simulink model "Expremental_work"  (R2020a)
settings: Solver=VariableStepAuto  StartTime=0.0  StopTime=10  RelTol=1e-3
values from neighbouring files (symbols this model uses):
  Ts = 0.02    [circle.m]
undefined symbols (not defined in the file or in its folder): a, sigbuilder_block
libraries: simulink x1
settings Model: Creator=Mostafa Mahmoud  LastModifiedBy=Mostafa Mahmoud

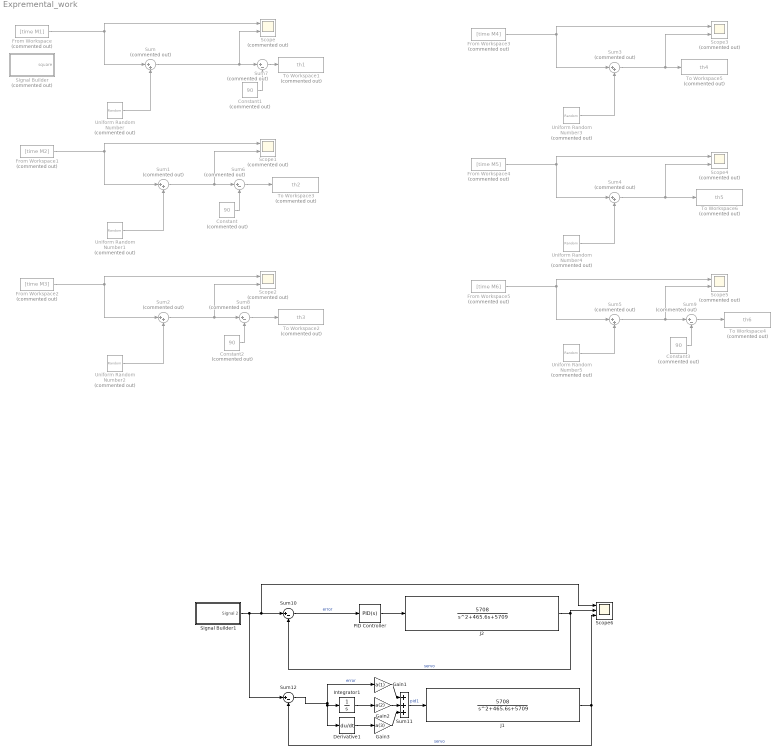
== system Expremental_work ==
  Constant{,1..3} (4 alike) : Constant  Commented=on  Value=90
  Derivative1 : Derivative
  From Workspace : FromWorkspace  Commented=on  VariableName=[time M1]  SampleTime=Ts
  From Workspace1 : FromWorkspace  Commented=on  VariableName=[time M2]  SampleTime=Ts
  From Workspace2 : FromWorkspace  Commented=on  VariableName=[time M3]  SampleTime=Ts
  From Workspace3 : FromWorkspace  Commented=on  VariableName=[time M4]  SampleTime=Ts
  From Workspace4 : FromWorkspace  Commented=on  VariableName=[time M5]  SampleTime=Ts
  From Workspace5 : FromWorkspace  Commented=on  VariableName=[time M6]  SampleTime=Ts
  Gain1 : Gain  Gain=a(1)
  Gain2 : Gain  Gain=a(2)
  Gain3 : Gain  Gain=a(3)
  Integrator1 : Integrator
  J1 : TransferFcn  Numerator=[5708]  Denominator=[1 465.6 5709]
  J2 : TransferFcn  Numerator=[5708]  Denominator=[1 465.6 5709]
  PID Controller : simulink/Continuous/PID Controller  Controller=PID  Form=Parallel  TimeDomain=Continuous-time  UseExternalTs=off  SampleTime=-1  IntegratorMethod=Forward Euler  FilterMethod=Forward Euler  ControllerParametersSource=internal  P=1.35854081151269  I=32.722901999271  D=-0.000923708182318546  UseFilter=on  N=26.187132412545  TunerSelectOption=Transfer Function Based (PID Tuner App)  InitialConditionSource=internal  InitialConditionForIntegrator=0  InitialConditionForFilter=0  DifferentiatorICPrevScaledInput=0  ExternalReset=none  TrackingMode=off  Kt=1  LimitOutput=on  UpperSaturationLimit=255  LowerSaturationLimit=0  LinearizeAsGain=on  AntiWindupMode=none  Kb=1  POutMin=[]  POutMax=[]  IOutMin=[]  IOutMax=[]  DOutMin=[]  DOutMax=[]  NOutMin=[]  NOutMax=[]  SumOutMin=[]  SumOutMax=[]  SaturationOutMin=[]  SaturationOutMax=[]  PParamMin=[]  PParamMax=[]  IParamMin=[]  IParamMax=[]  DParamMin=[]  DParamMax=[]  NParamMin=[]  NParamMax=[]  KbParamMin=[]  KbParamMax=[]  KtParamMin=[]  KtParamMax=[]  KbOutMin=[]  KbOutMax=[]  KtOutMin=[]  KtOutMax=[]  IntegratorOutMin=[]  IntegratorOutMax=[]  FilterOutMin=[]  FilterOutMax=[]  SumI1OutMin=[]  SumI1OutMax=[]  SumI2OutMin=[]  SumI2OutMax=[]  SumI3OutMin=[]  SumI3OutMax=[]  SumI4OutMin=[]  SumI4OutMax=[]  SumDOutMin=[]  SumDOutMax=[]  DifferentiatorOutMin=[]  DifferentiatorOutMax=[]  FilterDiffOutCoefMin=[]  FilterDiffOutCoefMax=[]  ReciprocalOutMin=[]  ReciprocalOutMax=[]  SumDenOutMin=[]  SumDenOutMax=[]  SumNumOutMin=[]  SumNumOutMax=[]  DivideOutMin=[]  DivideOutMax=[]  UdiffTsProdOutMin=[]  UdiffTsProdOutMax=[]  NTsProdOutMin=[]  NTsProdOutMax=[]  UintegralTsProdOutMin=[]  UintegralTsProdOutMax=[]  UngainTsProdOutMin=[]  UngainTsProdOutMax=[]  IntegratorContinuousStateAttributes=''  IntegratorStateMustResolveToSignalObject=off  IntegratorRTWStateStorageClass=Auto  FilterContinuousStateAttributes=''  FilterStateMustResolveToSignalObject=off  FilterRTWStateStorageClass=Auto  ParallelPVariant=InternalParameters  IdealPVariant=Disabled  IVariant=InternalParameters  DVariant=InternalParameters  IntegratorVariant=Continuous  SatVariant=Enabled  AWVariant=Passthrough  PCopyVariant=Disabled  TRVariant=Disabled  FdbkBlocksVariant=Forward  IdealPFdbkVariant=Disabled  SatFdbkVariant=Disabled  DerivativeFilterVariant=ContFilter  NVariant=InternalParameters  NCopyVariant=Disabled  FilterICVariant=InternalICsFilter  IntegratorICVariant=InternalICs  ExternalResetVariant=Disabled  TRSumVariant=Passthrough  SumFdbkVariant=Disabled  SumVariant=Sum_PID  TsampFilterVariant=InternalTs  TsampNgainVariant=Passthrough  TsampIntegralVariant=Passthrough
  Scope{,1..5} (6 alike) : Scope  Commented=on  NumInputPorts=2
  Scope6 : Scope  NumInputPorts=3
  Signal Builder : Subsystem  Tag=STV Subsys  Commented=on  LoadFcn=sigbuilder_block('load');  StartFcn=sigbuilder_block('start');  StopFcn=sigbuilder_block('stop');  ClipboardFcn=sigbuilder_block('clipboard');  mask(Sigbuilder block){tuvar=[0:10]}
      mask help: Simulink:masks:SigbuilderBlock_MD
      mask init:
      | if ~strcmp(get_param(bdroot(gcbh),'SimulationStatus'),'stopped') tuvar = sigbuilder_block('maskInit'); end
      settings: CopyFcn=sigbuilder_block('copy');  DeleteFcn=sigbuilder_block('delete');  ModelCloseFcn=sigbuilder_block('modelClose');  PreSaveFcn=sigbuilder_block('preSave');  PauseFcn=sigbuilder_block('pause');  ContinueFcn=sigbuilder_block('continue');  NameChangeFcn=sigbuilder_block('namechange');  OpenFcn=sigbuilder_block('open',[5.4 30 1141.2 522.6 ]);  CloseFcn=sigbuilder_block('close');
      mask Display: plot(0, 0, 100, 100,[2, 2, 32, 32, 2], [68, 8, 8, 68, 68],[32, 2], [38, 38], [32, 19, 2],[53, 60, 44], [32, 17, 17, 2],[16, 16, 31, 31]);txt = getActiveGroup(gcbh);text(2, 100, txt,'verticalAlignment', 'top');
  Signal Builder1 : Subsystem  Tag=STV Subsys  LoadFcn=sigbuilder_block('load');  StartFcn=sigbuilder_block('start');  StopFcn=sigbuilder_block('stop');  ClipboardFcn=sigbuilder_block('clipboard');  mask(Sigbuilder block){tuvar=[0:10]}
      mask help: Simulink:masks:SigbuilderBlock_MD
      mask init:
      | if ~strcmp(get_param(bdroot(gcbh),'SimulationStatus'),'stopped') tuvar = sigbuilder_block('maskInit'); end
      settings: CopyFcn=sigbuilder_block('copy');  DeleteFcn=sigbuilder_block('delete');  ModelCloseFcn=sigbuilder_block('modelClose');  PreSaveFcn=sigbuilder_block('preSave');  PauseFcn=sigbuilder_block('pause');  ContinueFcn=sigbuilder_block('continue');  NameChangeFcn=sigbuilder_block('namechange');  OpenFcn=sigbuilder_block('open',[437.6 199.2 550.4 400 ]);  CloseFcn=sigbuilder_block('close');
      mask Display: plot(0, 0, 100, 100,[2, 2, 32, 32, 2], [68, 8, 8, 68, 68],[32, 2], [38, 38], [32, 19, 2],[53, 60, 44], [32, 17, 17, 2],[16, 16, 31, 31]);txt = getActiveGroup(gcbh);text(2, 100, txt,'verticalAlignment', 'top');
  Sum{,1..5} (6 alike) : Sum  Commented=on  Inputs=|++
  Sum10 : Sum  Inputs=|+-
  Sum11 : Sum  Inputs=+++
  Sum12 : Sum  Inputs=|+-
  Sum{6..9} (4 alike) : Sum  Commented=on  Inputs=|+-
  To Workspace1 : ToWorkspace  Commented=on  VariableName=th1  SampleTime=1
  To Workspace2 : ToWorkspace  Commented=on  VariableName=th3  SampleTime=1
  To Workspace3 : ToWorkspace  Commented=on  VariableName=th2  SampleTime=1
  To Workspace4 : ToWorkspace  Commented=on  VariableName=th6  SampleTime=1
  To Workspace5 : ToWorkspace  Commented=on  VariableName=th4  SampleTime=1
  To Workspace6 : ToWorkspace  Commented=on  VariableName=th5  SampleTime=1
  Uniform Random Number{,1..5} (6 alike) : UniformRandomNumber  Commented=on  Minimum=-0.1  Maximum=0.1  SampleTime=Ts
  wires:
  Uniform Random Number/1 -> Sum/2
  From Workspace/1 -> Sum/1, Scope/1
  From Workspace1/1 -> Scope1/1, Sum1/1
  Uniform Random Number1/1 -> Sum1/2
  Sum1/1 -> Sum6/1, Scope1/2
  Uniform Random Number2/1 -> Sum2/2
  From Workspace2/1 -> Scope2/1, Sum2/1
  Uniform Random Number3/1 -> Sum3/2
  Sum3/1 -> To Workspace5/1, Scope3/2
  From Workspace3/1 -> Scope3/1, Sum3/1
  From Workspace4/1 -> Scope4/1, Sum4/1
  Sum4/1 -> To Workspace6/1, Scope4/2
  Uniform Random Number4/1 -> Sum4/2
  Uniform Random Number5/1 -> Sum5/2
  From Workspace5/1 -> Scope5/1, Sum5/1
  Constant/1 -> Sum6/2
  Sum6/1 -> To Workspace3/1
  Sum/1 -> Sum7/1, Scope/2
  Constant1/1 -> Sum7/2
  Sum7/1 -> To Workspace1/1
  Sum2/1 -> Scope2/2, Sum8/1
  Constant2/1 -> Sum8/2
  Sum8/1 -> To Workspace2/1
  Sum5/1 -> Sum9/1, Scope5/2
  Constant3/1 -> Sum9/2
  Sum9/1 -> To Workspace4/1
  Sum10/1 -> PID Controller/1  "error"
  PID Controller/1 -> J2/1
  J2/1 -> Sum10/2, Scope6/2  "servo"
  Signal Builder1/1(Signal 2) -> Sum12/1, Scope6/1, Sum10/1
  Gain1/1 -> Sum11/1
  Sum11/1 -> J1/1  "pid1"
  Gain3/1 -> Sum11/3
  Derivative1/1 -> Gain3/1
  Sum12/1 -> Derivative1/1, Integrator1/1, Gain1/1  "error"
  Integrator1/1 -> Gain2/1
  Gain2/1 -> Sum11/2
  J1/1 -> Scope6/3, Sum12/2  "servo"

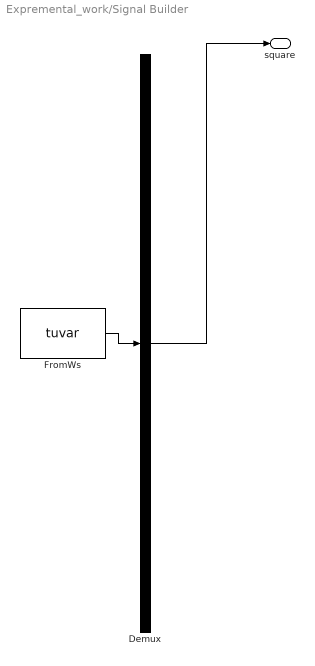
== system Expremental_work/Signal Builder ==
  Demux : Demux  Tag=STV Demux  Outputs=1
      settings: DisplayOption=none
  FromWs : FromWorkspace  Tag=STV FromWs  VariableName=tuvar
      SigBuilderData=|
      | common.afterFinalStr = 'Extrapolate'
      | common.sampleTime = 0
      | dataSet.timeRange = [0 10]
      | dataSet.name = 'Group 1'
      | sbobj.Groups.Name = 'Group 1'
      | sbobj.Groups.Signals.Name = 'square'
      | sbobj.Groups.Signals.XData = [0 1 1 2 2 3 3 4 4 5 5 6 6 7 7 8 8 9 9 10]
      | sbobj.Groups.Signals.YData = [135 135 45 45 135 135 45 45 135 135 45 45 135 135 45 45 135 135 45 45]
  square : Outport  Tag=STV Outport
  wires:
  FromWs/1 -> Demux/1
  Demux/1 -> square/1

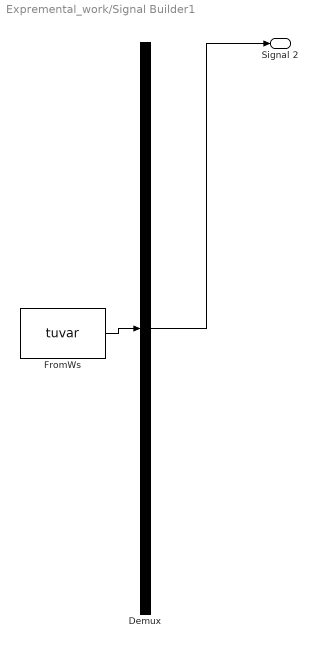
== system Expremental_work/Signal Builder1 ==
  Demux : Demux  Tag=STV Demux  Outputs=1
      settings: DisplayOption=none
  FromWs : FromWorkspace  Tag=STV FromWs  VariableName=tuvar
      SigBuilderData=|
      | common.afterFinalStr = 'Extrapolate'
      | common.sampleTime = 0
      | dataSet.timeRange = [0 10]
      | dataSet.name = 'Group 1'
      | sbobj.Groups.Name = 'Group 1'
      | sbobj.Groups.Signals.Name = 'Signal 2'
      | sbobj.Groups.Signals.XData = [0 5 5 10]
      | sbobj.Groups.Signals.YData = [0 0 90 90]
  Signal 2 : Outport  Tag=STV Outport
  wires:
  FromWs/1 -> Demux/1
  Demux/1 -> Signal 2/1
